simulink model "RavenSystem"  (R2025b)
settings: Solver=VariableStepAuto  StartTime=0.0  StopTime=10.0  RelTol=1e-3
(part 2 of 2)

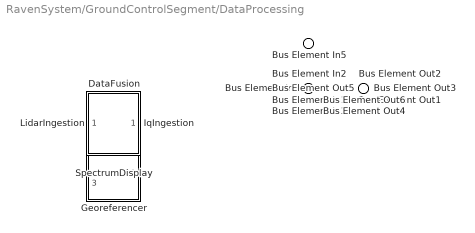
== system RavenSystem/GroundControlSegment/DataProcessing ==
  Bus Element In5 : Inport  PortName=InBus
  Bus Element In1 : Inport  Port=2  PortName=IqStreamIn
  Bus Element In2 : Inport  Port=3  PortName=LidarDataIn
  Bus Element In3 : Inport  Port=4  PortName=IqStreamIn1
  Bus Element In4 : Inport  Port=5  PortName=LidarDataIn1
  DataFusion : Subsystem
      settings: PortSchema="{\"entries\":[{\"content\":{\"headerSize\":26,\"margin\":15,\"minimumSpacing\":25,\"sides\":[{\"content\":{\"connectorIds\":[\"In1\",\"In2\"]},\"type\":\"ConnectorPlacement.EquallySpacedRectSide\",\"uuid\":\"d227efd3-a579-41d6-b0ed-0ed28488032b\"},{\"content\":{\"connectorIds\":[\"Out1\"],\"side\":\"RIGHT\"},\"type\":\"ConnectorPlacement.EquallySpacedRectSide\",\"uuid\":\"95cb1b72-47dc-4890-bf9d-9edbae3db4aa\"},{\"content\":{\"side\":\"TOP\"},\"type\":\"ConnectorPlacement.EquallySpacedRectSide\",\"uuid\":\"15e0707d-618d-4be9-b8fd-b627fcfb261f\"}]},\"type\":\"ConnectorPlacement.EquallySpacedConnector\",\"uuid\":\"3c106411-bdfa-4db9-bf7b-e312ca1d0dec\"}],\"packageUris\":[\"http://schema.mathworks.com/mf0/Connector/R2020b\"],\"version\":\"1.0\"}"
  Georeferencer : Subsystem
      settings: PortSchema="{\"entries\":[{\"content\":{\"headerSize\":26,\"margin\":15,\"minimumSpacing\":25,\"sides\":[{\"content\":{\"connectorIds\":[\"In1\",\"In2\",\"In3\"]},\"type\":\"ConnectorPlacement.EquallySpacedRectSide\",\"uuid\":\"d227efd3-a579-41d6-b0ed-0ed28488032b\"},{\"content\":{\"connectorIds\":[\"Out1\",\"Out2\"],\"side\":\"RIGHT\"},\"type\":\"ConnectorPlacement.EquallySpacedRectSide\",\"uuid\":\"95cb1b72-47dc-4890-bf9d-9edbae3db4aa\"},{\"content\":{\"side\":\"TOP\"},\"type\":\"ConnectorPlacement.EquallySpacedRectSide\",\"uuid\":\"15e0707d-618d-4be9-b8fd-b627fcfb261f\"}]},\"type\":\"ConnectorPlacement.EquallySpacedConnector\",\"uuid\":\"3c106411-bdfa-4db9-bf7b-e312ca1d0dec\"}],\"packageUris\":[\"http://schema.mathworks.com/mf0/Connector/R2020b\"],\"version\":\"1.0\"}"
  IqIngestion : Subsystem
      settings: PortSchema="{\"entries\":[{\"content\":{\"headerSize\":26,\"margin\":15,\"minimumSpacing\":25,\"sides\":[{\"content\":{\"connectorIds\":[\"In1\"]},\"type\":\"ConnectorPlacement.EquallySpacedRectSide\",\"uuid\":\"d227efd3-a579-41d6-b0ed-0ed28488032b\"},{\"content\":{\"connectorIds\":[\"Out1\"],\"side\":\"RIGHT\"},\"type\":\"ConnectorPlacement.EquallySpacedRectSide\",\"uuid\":\"95cb1b72-47dc-4890-bf9d-9edbae3db4aa\"},{\"content\":{\"side\":\"TOP\"},\"type\":\"ConnectorPlacement.EquallySpacedRectSide\",\"uuid\":\"15e0707d-618d-4be9-b8fd-b627fcfb261f\"}]},\"type\":\"ConnectorPlacement.EquallySpacedConnector\",\"uuid\":\"3c106411-bdfa-4db9-bf7b-e312ca1d0dec\"}],\"packageUris\":[\"http://schema.mathworks.com/mf0/Connector/R2020b\"],\"version\":\"1.0\"}"
  LidarIngestion : Subsystem
      settings: PortSchema="{\"entries\":[{\"content\":{\"headerSize\":26,\"margin\":15,\"minimumSpacing\":25,\"sides\":[{\"content\":{\"connectorIds\":[\"In1\"]},\"type\":\"ConnectorPlacement.EquallySpacedRectSide\",\"uuid\":\"d227efd3-a579-41d6-b0ed-0ed28488032b\"},{\"content\":{\"connectorIds\":[\"Out1\"],\"side\":\"RIGHT\"},\"type\":\"ConnectorPlacement.EquallySpacedRectSide\",\"uuid\":\"95cb1b72-47dc-4890-bf9d-9edbae3db4aa\"},{\"content\":{\"side\":\"TOP\"},\"type\":\"ConnectorPlacement.EquallySpacedRectSide\",\"uuid\":\"15e0707d-618d-4be9-b8fd-b627fcfb261f\"}]},\"type\":\"ConnectorPlacement.EquallySpacedConnector\",\"uuid\":\"3c106411-bdfa-4db9-bf7b-e312ca1d0dec\"}],\"packageUris\":[\"http://schema.mathworks.com/mf0/Connector/R2020b\"],\"version\":\"1.0\"}"
  SpectrumDisplay : Subsystem
      settings: PortSchema="{\"entries\":[{\"content\":{\"headerSize\":26,\"margin\":15,\"minimumSpacing\":25,\"sides\":[{\"content\":{\"connectorIds\":[\"In1\"]},\"type\":\"ConnectorPlacement.EquallySpacedRectSide\",\"uuid\":\"d227efd3-a579-41d6-b0ed-0ed28488032b\"},{\"content\":{\"connectorIds\":[\"Out1\"],\"side\":\"RIGHT\"},\"type\":\"ConnectorPlacement.EquallySpacedRectSide\",\"uuid\":\"95cb1b72-47dc-4890-bf9d-9edbae3db4aa\"},{\"content\":{\"side\":\"TOP\"},\"type\":\"ConnectorPlacement.EquallySpacedRectSide\",\"uuid\":\"15e0707d-618d-4be9-b8fd-b627fcfb261f\"}]},\"type\":\"ConnectorPlacement.EquallySpacedConnector\",\"uuid\":\"3c106411-bdfa-4db9-bf7b-e312ca1d0dec\"}],\"packageUris\":[\"http://schema.mathworks.com/mf0/Connector/R2020b\"],\"version\":\"1.0\"}"
  Bus Element Out1 : Outport  PortName=GeoreferencedRfOut
  Bus Element Out2 : Outport  Port=2  PortName=FusedDataProductOut
  Bus Element Out3 : Outport  Port=3  PortName=SpectrumDisplayOut
  Bus Element Out4 : Outport  Port=4  PortName=GeoreferencedRfOut1
  Bus Element Out5 : Outport  Port=5  PortName=FusedDataProductOut1
  Bus Element Out6 : Outport  Port=6  PortName=SpectrumDisplayOut1

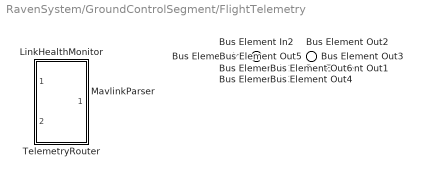
== system RavenSystem/GroundControlSegment/FlightTelemetry ==
  Bus Element In1 : Inport  PortName=MavlinkCmdIn
  Bus Element In2 : Inport  Port=2  PortName=DataLinkIn
  Bus Element In3 : Inport  Port=3  PortName=MavlinkCmdIn1
  Bus Element In4 : Inport  Port=4  PortName=DataLinkIn1
  LinkHealthMonitor : Subsystem
      settings: PortSchema="{\"entries\":[{\"content\":{\"headerSize\":26,\"margin\":15,\"minimumSpacing\":25,\"sides\":[{\"content\":{\"connectorIds\":[\"In1\"]},\"type\":\"ConnectorPlacement.EquallySpacedRectSide\",\"uuid\":\"d227efd3-a579-41d6-b0ed-0ed28488032b\"},{\"content\":{\"connectorIds\":[\"Out1\"],\"side\":\"RIGHT\"},\"type\":\"ConnectorPlacement.EquallySpacedRectSide\",\"uuid\":\"95cb1b72-47dc-4890-bf9d-9edbae3db4aa\"},{\"content\":{\"side\":\"TOP\"},\"type\":\"ConnectorPlacement.EquallySpacedRectSide\",\"uuid\":\"15e0707d-618d-4be9-b8fd-b627fcfb261f\"}]},\"type\":\"ConnectorPlacement.EquallySpacedConnector\",\"uuid\":\"3c106411-bdfa-4db9-bf7b-e312ca1d0dec\"}],\"packageUris\":[\"http://schema.mathworks.com/mf0/Connector/R2020b\"],\"version\":\"1.0\"}"
  MavlinkParser : Subsystem
      settings: PortSchema="{\"entries\":[{\"content\":{\"headerSize\":26,\"margin\":15,\"minimumSpacing\":25,\"sides\":[{\"content\":{\"connectorIds\":[\"In1\"]},\"type\":\"ConnectorPlacement.EquallySpacedRectSide\",\"uuid\":\"d227efd3-a579-41d6-b0ed-0ed28488032b\"},{\"content\":{\"connectorIds\":[\"Out1\"],\"side\":\"RIGHT\"},\"type\":\"ConnectorPlacement.EquallySpacedRectSide\",\"uuid\":\"95cb1b72-47dc-4890-bf9d-9edbae3db4aa\"},{\"content\":{\"side\":\"TOP\"},\"type\":\"ConnectorPlacement.EquallySpacedRectSide\",\"uuid\":\"15e0707d-618d-4be9-b8fd-b627fcfb261f\"}]},\"type\":\"ConnectorPlacement.EquallySpacedConnector\",\"uuid\":\"3c106411-bdfa-4db9-bf7b-e312ca1d0dec\"}],\"packageUris\":[\"http://schema.mathworks.com/mf0/Connector/R2020b\"],\"version\":\"1.0\"}"
  TelemetryRouter : Subsystem
      settings: PortSchema="{\"entries\":[{\"content\":{\"headerSize\":26,\"margin\":15,\"minimumSpacing\":25,\"sides\":[{\"content\":{\"connectorIds\":[\"In1\",\"In2\"]},\"type\":\"ConnectorPlacement.EquallySpacedRectSide\",\"uuid\":\"d227efd3-a579-41d6-b0ed-0ed28488032b\"},{\"content\":{\"connectorIds\":[\"Out1\"],\"side\":\"RIGHT\"},\"type\":\"ConnectorPlacement.EquallySpacedRectSide\",\"uuid\":\"95cb1b72-47dc-4890-bf9d-9edbae3db4aa\"},{\"content\":{\"side\":\"TOP\"},\"type\":\"ConnectorPlacement.EquallySpacedRectSide\",\"uuid\":\"15e0707d-618d-4be9-b8fd-b627fcfb261f\"}]},\"type\":\"ConnectorPlacement.EquallySpacedConnector\",\"uuid\":\"3c106411-bdfa-4db9-bf7b-e312ca1d0dec\"}],\"packageUris\":[\"http://schema.mathworks.com/mf0/Connector/R2020b\"],\"version\":\"1.0\"}"
  Bus Element Out1 : Outport  PortName=TelemetryOut
  Bus Element Out2 : Outport  Port=2  PortName=LinkHealthOut
  Bus Element Out3 : Outport  Port=3  PortName=DataLinkOut
  Bus Element Out4 : Outport  Port=4  PortName=TelemetryOut1
  Bus Element Out5 : Outport  Port=5  PortName=LinkHealthOut1
  Bus Element Out6 : Outport  Port=6  PortName=DataLinkOut1

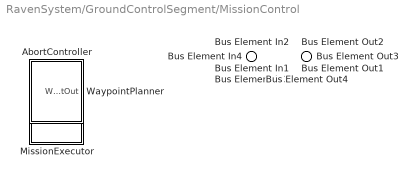
== system RavenSystem/GroundControlSegment/MissionControl ==
  Bus Element In1 : Inport  PortName=TelemetryIn
  Bus Element In2 : Inport  Port=2  PortName=MissionStatusIn
  Bus Element In3 : Inport  Port=3  PortName=TelemetryIn1
  Bus Element In4 : Inport  Port=4  PortName=MissionStatusIn1
  AbortController : Subsystem
      settings: PortSchema="{\"entries\":[{\"content\":{\"headerSize\":26,\"margin\":15,\"minimumSpacing\":25,\"sides\":[{\"content\":{\"connectorIds\":[\"In1\"]},\"type\":\"ConnectorPlacement.EquallySpacedRectSide\",\"uuid\":\"d227efd3-a579-41d6-b0ed-0ed28488032b\"},{\"content\":{\"connectorIds\":[\"Out1\"],\"side\":\"RIGHT\"},\"type\":\"ConnectorPlacement.EquallySpacedRectSide\",\"uuid\":\"95cb1b72-47dc-4890-bf9d-9edbae3db4aa\"},{\"content\":{\"side\":\"TOP\"},\"type\":\"ConnectorPlacement.EquallySpacedRectSide\",\"uuid\":\"15e0707d-618d-4be9-b8fd-b627fcfb261f\"}]},\"type\":\"ConnectorPlacement.EquallySpacedConnector\",\"uuid\":\"3c106411-bdfa-4db9-bf7b-e312ca1d0dec\"}],\"packageUris\":[\"http://schema.mathworks.com/mf0/Connector/R2020b\"],\"version\":\"1.0\"}"
  MissionExecutor : Subsystem
      settings: PortSchema="{\"entries\":[{\"content\":{\"headerSize\":26,\"margin\":15,\"minimumSpacing\":25,\"sides\":[{\"content\":{\"connectorIds\":[\"In1\"]},\"type\":\"ConnectorPlacement.EquallySpacedRectSide\",\"uuid\":\"d227efd3-a579-41d6-b0ed-0ed28488032b\"},{\"content\":{\"connectorIds\":[\"Out1\",\"Out2\"],\"side\":\"RIGHT\"},\"type\":\"ConnectorPlacement.EquallySpacedRectSide\",\"uuid\":\"95cb1b72-47dc-4890-bf9d-9edbae3db4aa\"},{\"content\":{\"side\":\"TOP\"},\"type\":\"ConnectorPlacement.EquallySpacedRectSide\",\"uuid\":\"15e0707d-618d-4be9-b8fd-b627fcfb261f\"}]},\"type\":\"ConnectorPlacement.EquallySpacedConnector\",\"uuid\":\"3c106411-bdfa-4db9-bf7b-e312ca1d0dec\"}],\"packageUris\":[\"http://schema.mathworks.com/mf0/Connector/R2020b\"],\"version\":\"1.0\"}"
  WaypointPlanner : Subsystem
      settings: PortSchema="{\"entries\":[{\"content\":{\"headerSize\":26,\"margin\":15,\"minimumSpacing\":25,\"sides\":[{\"content\":{},\"type\":\"ConnectorPlacement.EquallySpacedRectSide\",\"uuid\":\"d227efd3-a579-41d6-b0ed-0ed28488032b\"},{\"content\":{\"connectorIds\":[\"Out1\"],\"side\":\"RIGHT\"},\"type\":\"ConnectorPlacement.EquallySpacedRectSide\",\"uuid\":\"95cb1b72-47dc-4890-bf9d-9edbae3db4aa\"},{\"content\":{\"side\":\"TOP\"},\"type\":\"ConnectorPlacement.EquallySpacedRectSide\",\"uuid\":\"15e0707d-618d-4be9-b8fd-b627fcfb261f\"}]},\"type\":\"ConnectorPlacement.EquallySpacedConnector\",\"uuid\":\"3c106411-bdfa-4db9-bf7b-e312ca1d0dec\"}],\"packageUris\":[\"http://schema.mathworks.com/mf0/Connector/R2020b\"],\"version\":\"1.0\"}"
  Bus Element Out1 : Outport  PortName=MavlinkCmdOut
  Bus Element Out2 : Outport  Port=2  PortName=AbortCmdOut
  Bus Element Out3 : Outport  Port=3  PortName=MavlinkCmdOut1
  Bus Element Out4 : Outport  Port=4  PortName=AbortCmdOut1

== system RavenSystem/AerialVehicleSegment/FlightComputer/GpsDaemon ==
  Bus Element Out1 : Outport  PortName=GpsCoordOut

== system RavenSystem/AerialVehicleSegment/FlightComputer/LidarDriver ==
  Bus Element In1 : Inport  PortName=RawScanIn
  Bus Element Out1 : Outport  PortName=PointCloudOut

== system RavenSystem/AerialVehicleSegment/FlightComputer/MavlinkBridge ==
  Bus Element In1 : Inport  PortName=UartMavlinkIn
  Bus Element In2 : Inport  Port=2  PortName=WifiMavlinkIn
  Bus Element Out1 : Outport  PortName=WifiMavlinkOut
  Bus Element Out2 : Outport  Port=2  PortName=UartMavlinkOut

== system RavenSystem/AerialVehicleSegment/FlightComputer/RaspberryPi5 ==
  Bus Element Out1 : Outport  PortName=ComputeOut

== system RavenSystem/AerialVehicleSegment/FlightComputer/RtlTcpServer ==
  Bus Element In1 : Inport  PortName=IqDataIn
  Bus Element Out1 : Outport  PortName=IqStreamOut

== system RavenSystem/AerialVehicleSegment/FlightComputer/UavDaemon ==
  Bus Element In1 : Inport  PortName=ComputeIn
  Bus Element In2 : Inport  Port=2  PortName=GpsTagIn
  Bus Element Out1 : Outport  PortName=MavlinkBridgeOut
  Bus Element Out2 : Outport  Port=2  PortName=RtlTcpOut
  Bus Element Out3 : Outport  Port=3  PortName=LidarLogOut

== system RavenSystem/AerialVehicleSegment/FlightControl/ArduPilot ==
  Bus Element In1 : Inport  PortName=ImuIn
  Bus Element In2 : Inport  Port=2  PortName=BaroIn
  Bus Element In3 : Inport  Port=3  PortName=GpsIn
  Bus Element In4 : Inport  Port=4  PortName=WaypointIn
  Bus Element Out1 : Outport  PortName=AttitudeCmdOut

== system RavenSystem/AerialVehicleSegment/FlightControl/AttitudeController ==
  Bus Element In1 : Inport  PortName=AttitudeCmdIn
  Bus Element Out1 : Outport  PortName=MotorCmdOut

== system RavenSystem/AerialVehicleSegment/FlightControl/Pixhawk6cMini ==
  Bus Element In1 : Inport  PortName=MavlinkIn
  Bus Element Out1 : Outport  PortName=MavlinkOut
  Bus Element Out2 : Outport  Port=2  PortName=ImuDataOut
  Bus Element Out3 : Outport  Port=3  PortName=BaroDataOut
  Bus Element Out4 : Outport  Port=4  PortName=GpsDataOut

== system RavenSystem/AerialVehicleSegment/FlightControl/WaypointExecutor ==
  Bus Element In1 : Inport  PortName=MavlinkCmdIn
  Bus Element Out1 : Outport  PortName=WaypointOut

== system RavenSystem/AerialVehicleSegment/Lidar/LidarUsbInterface ==
  Bus Element In1 : Inport  PortName=RawScanIn
  Bus Element Out1 : Outport  PortName=PointCloudOut

== system RavenSystem/AerialVehicleSegment/Lidar/RplidarA1M8 ==
  Bus Element Out1 : Outport  PortName=RawScanOut

== system RavenSystem/AerialVehicleSegment/Power/Bec5V ==
  Bus Element In1 : Inport  PortName=UnregulatedIn
  Bus Element Out1 : Outport  PortName=RegulatedPwrOut

== system RavenSystem/AerialVehicleSegment/Power/LipoBattery4S ==
  Bus Element Out1 : Outport  PortName=RawPowerOut

== system RavenSystem/AerialVehicleSegment/Power/PowerDistributionBoard ==
  Bus Element In1 : Inport  PortName=RawPowerIn
  Bus Element Out1 : Outport  PortName=FlightPowerOut
  Bus Element Out2 : Outport  Port=2  PortName=BecPowerOut

== system RavenSystem/AerialVehicleSegment/Propulsion/Esc1 ==
  Bus Element In1 : Inport  PortName=PwmCmdIn
  Bus Element In2 : Inport  Port=2  PortName=PowerIn
  Bus Element Out1 : Outport  PortName=PwmOut

== system RavenSystem/AerialVehicleSegment/Propulsion/Esc2 ==
  Bus Element In1 : Inport  PortName=PwmCmdIn
  Bus Element In2 : Inport  Port=2  PortName=PowerIn
  Bus Element Out1 : Outport  PortName=PwmOut

== system RavenSystem/AerialVehicleSegment/Propulsion/Esc3 ==
  Bus Element In1 : Inport  PortName=PwmCmdIn
  Bus Element In2 : Inport  Port=2  PortName=PowerIn
  Bus Element Out1 : Outport  PortName=PwmOut

== system RavenSystem/AerialVehicleSegment/Propulsion/Esc4 ==
  Bus Element In1 : Inport  PortName=PwmCmdIn
  Bus Element In2 : Inport  Port=2  PortName=PowerIn
  Bus Element Out1 : Outport  PortName=PwmOut

== system RavenSystem/AerialVehicleSegment/Propulsion/Motor1 ==
  Bus Element In1 : Inport  PortName=PwmIn
  Bus Element In2 : Inport  Port=2  PortName=PowerIn
  Bus Element Out1 : Outport  PortName=ShaftOut

== system RavenSystem/AerialVehicleSegment/Propulsion/Motor2 ==
  Bus Element In1 : Inport  PortName=PwmIn
  Bus Element In2 : Inport  Port=2  PortName=PowerIn
  Bus Element Out1 : Outport  PortName=ShaftOut

== system RavenSystem/AerialVehicleSegment/Propulsion/Motor3 ==
  Bus Element In1 : Inport  PortName=PwmIn
  Bus Element In2 : Inport  Port=2  PortName=PowerIn
  Bus Element Out1 : Outport  PortName=ShaftOut

== system RavenSystem/AerialVehicleSegment/Propulsion/Motor4 ==
  Bus Element In1 : Inport  PortName=PwmIn
  Bus Element In2 : Inport  Port=2  PortName=PowerIn
  Bus Element Out1 : Outport  PortName=ShaftOut

== system RavenSystem/AerialVehicleSegment/Propulsion/Propeller1 ==
  Bus Element In1 : Inport  PortName=ShaftIn
  Bus Element Out1 : Outport  PortName=ThrustOut

== system RavenSystem/AerialVehicleSegment/Propulsion/Propeller2 ==
  Bus Element In1 : Inport  PortName=ShaftIn
  Bus Element Out1 : Outport  PortName=ThrustOut

== system RavenSystem/AerialVehicleSegment/Propulsion/Propeller3 ==
  Bus Element In1 : Inport  PortName=ShaftIn
  Bus Element Out1 : Outport  PortName=ThrustOut

== system RavenSystem/AerialVehicleSegment/Propulsion/Propeller4 ==
  Bus Element In1 : Inport  PortName=ShaftIn
  Bus Element Out1 : Outport  PortName=ThrustOut

== system RavenSystem/AerialVehicleSegment/RfSdr/RtlSdrV4 ==
  Bus Element In1 : Inport  PortName=RfSignalIn
  Bus Element Out1 : Outport  PortName=IqDataOut

== system RavenSystem/AerialVehicleSegment/RfSdr/SmaAntenna ==
  Bus Element Out1 : Outport  PortName=RfSignalOut

== system RavenSystem/AerialVehicleSegment/RfSdr/UsbInterface ==
  Bus Element In1 : Inport  PortName=IqDataIn
  Bus Element Out1 : Outport  PortName=IqStreamOut

== system RavenSystem/AerialVehicleSegment/Structures/AntennaMount ==
  Bus Element Out1 : Outport  PortName=AntennaMountOut

== system RavenSystem/AerialVehicleSegment/Structures/F450Frame ==
  Bus Element Out1 : Outport  PortName=StructuralSupportOut

== system RavenSystem/AerialVehicleSegment/Structures/LandingGear ==
  Bus Element Out1 : Outport  PortName=GroundSupportOut

== system RavenSystem/AerialVehicleSegment/Structures/PayloadMount ==
  Bus Element In1 : Inport  PortName=StructuralSupportIn
  Bus Element Out1 : Outport  PortName=PayloadMountOut

== system RavenSystem/GroundControlSegment/DataProcessing/DataFusion ==
  Bus Element In1 : Inport  PortName=GeoreferencedRfIn
  Bus Element In2 : Inport  Port=2  PortName=GeoreferencedLiIn
  Bus Element Out1 : Outport  PortName=FusedProductOut

== system RavenSystem/GroundControlSegment/DataProcessing/Georeferencer ==
  Bus Element In1 : Inport  PortName=SpectrumIn
  Bus Element In2 : Inport  Port=2  PortName=PointCloudIn
  Bus Element In3 : Inport  Port=3  PortName=GpsTagIn
  Bus Element Out1 : Outport  PortName=GeoreferencedRfOut
  Bus Element Out2 : Outport  Port=2  PortName=GeoreferencedLiOut

== system RavenSystem/GroundControlSegment/DataProcessing/IqIngestion ==
  Bus Element In1 : Inport  PortName=RawIqIn
  Bus Element Out1 : Outport  PortName=SpectrumSnapshotOut

== system RavenSystem/GroundControlSegment/DataProcessing/LidarIngestion ==
  Bus Element In1 : Inport  PortName=RawPointCloudIn
  Bus Element Out1 : Outport  PortName=TaggedCloudOut

== system RavenSystem/GroundControlSegment/DataProcessing/SpectrumDisplay ==
  Bus Element In1 : Inport  PortName=SpectrumIn
  Bus Element Out1 : Outport  PortName=DisplayOut

== system RavenSystem/GroundControlSegment/FlightTelemetry/LinkHealthMonitor ==
  Bus Element In1 : Inport  PortName=HeartbeatIn
  Bus Element Out1 : Outport  PortName=LinkStatusOut

== system RavenSystem/GroundControlSegment/FlightTelemetry/MavlinkParser ==
  Bus Element In1 : Inport  PortName=RawMavlinkIn
  Bus Element Out1 : Outport  PortName=ParsedTlmOut

== system RavenSystem/GroundControlSegment/FlightTelemetry/TelemetryRouter ==
  Bus Element In1 : Inport  PortName=TelemetryIn
  Bus Element In2 : Inport  Port=2  PortName=MavlinkCmdIn
  Bus Element Out1 : Outport  PortName=DataLinkOut

== system RavenSystem/GroundControlSegment/MissionControl/AbortController ==
  Bus Element In1 : Inport  PortName=TelemetryIn
  Bus Element Out1 : Outport  PortName=AbortCmdOut

== system RavenSystem/GroundControlSegment/MissionControl/MissionExecutor ==
  Bus Element In1 : Inport  PortName=WaypointListIn
  Bus Element Out1 : Outport  PortName=MavlinkCmdOut
  Bus Element Out2 : Outport  Port=2  PortName=MissionStatusOut

== system RavenSystem/GroundControlSegment/MissionControl/WaypointPlanner ==
  Bus Element Out1 : Outport  PortName=WaypointListOut
